simulink model "LinearniUpravljanje"  (R2018a)
settings: Solver=VariableStepAuto  StartTime=0.0  StopTime=15  RelTol=1e-3  EnableMultiTasking=on
values from neighbouring files (symbols this model uses):
  a11 = double(subs(diff(f1,wm),[wm id iq u1 mh],[wmn idn iqn u1n mhn]))    [Linearizacija.m]
  a12 = double(subs(diff(f1,id),[wm id iq u1 mh],[wmn idn iqn u1n mhn]))    [Linearizacija.m]
  a13 = double(subs(diff(f1,iq),[wm id iq u1 mh],[wmn idn iqn u1n mhn]))    [Linearizacija.m]
  a21 = double(subs(diff(f2,wm),[wm id iq u1 mh],[wmn idn iqn u1n mhn]))    [Linearizacija.m]
  a22 = double(subs(diff(f2,id),[wm id iq u1 mh],[wmn idn iqn u1n mhn]))    [Linearizacija.m]
  a23 = double(subs(diff(f2,iq),[wm id iq u1 mh],[wmn idn iqn u1n mhn]))    [Linearizacija.m]
  a31 = double(subs(diff(f3,wm),[wm id iq u1 mh],[wmn idn iqn u1n mhn]))    [Linearizacija.m]
  a32 = double(subs(diff(f3,id),[wm id iq u1 mh],[wmn idn iqn u1n mhn]))    [Linearizacija.m]
  a33 = double(subs(diff(f3,iq),[wm id iq u1 mh],[wmn idn iqn u1n mhn]))    [Linearizacija.m]
  b11 = double(subs(diff(f1,u1),[wm id iq u1 mh],[wmn idn iqn u1n mhn]))    [Linearizacija.m]
  b12 = double(subs(diff(f1,mh),[wm id iq u1 mh],[wmn idn iqn u1n mhn]))    [Linearizacija.m]
  b21 = double(subs(diff(f2,u1),[wm id iq u1 mh],[wmn idn iqn u1n mhn]))    [Linearizacija.m]
  b22 = double(subs(diff(f2,mh),[wm id iq u1 mh],[wmn idn iqn u1n mhn]))    [Linearizacija.m]
  b31 = double(subs(diff(f3,u1),[wm id iq u1 mh],[wmn idn iqn u1n mhn]))    [Linearizacija.m]
  b32 = double(subs(diff(f3,mh),[wm id iq u1 mh],[wmn idn iqn u1n mhn]))    [Linearizacija.m]
  idn = Odgovor(2)    [nominale.m]
  iqn = Odgovor(3)    [nominale.m]
  nn = 3000    [Podaci.m]    (also in Podaci.mat; nominale.m)
  u1n = Odgovor(1)    [nominale.m]
  wmn = nn*pi/30    (= 314.159265359)    [nominale.m]
libraries: simulink x1
settings Model: Creator=Bane  LastModifiedBy=lakim
settings DataIOCC: LimitDataPoints=on
settings OptimizationCC: LifeSpan=inf
settings DebuggingCC: AllowSymbolicDim=off  SFUnexpectedBacktrackingDiag=warning  SFNoUnconditionalDefaultTransitionDiag=warning  SFExecutionAtInitializationDiag=none
settings ModelReferenceCC: PropagateSignalLabelsOutOfModel=off
settings CodeAppCC: StateflowObjectComments=on
settings GRTTargetCC: TargetLangStandard=C89/C90 (ANSI)
settings ConfigComp: CovMetricSettings=dw  CovHtmlReporting=on  CovSaveCumulativeToWorkspaceVar=on  CovSaveSingleToWorkspaceVar=on  CovExternalEMLEnable=off

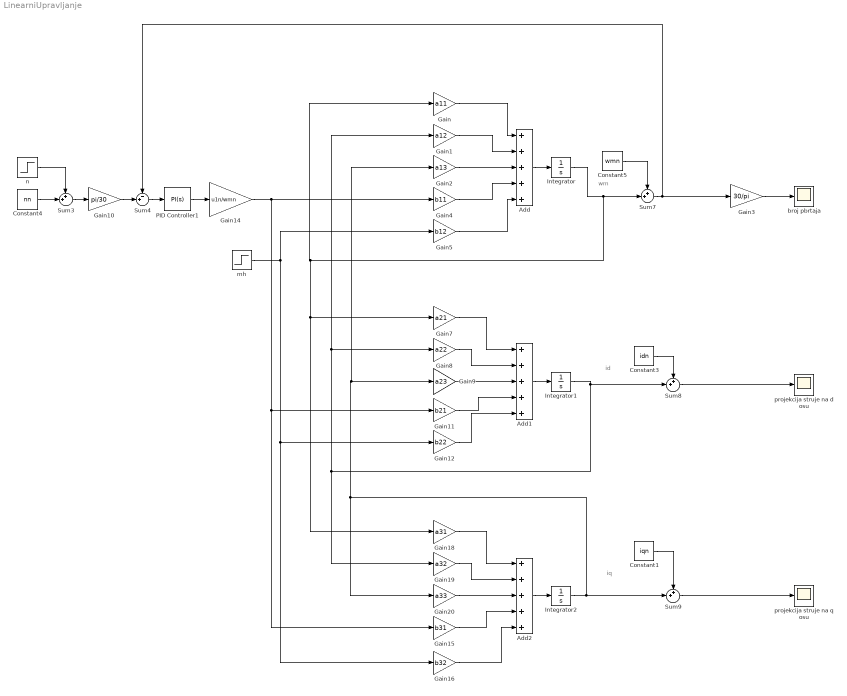
== system LinearniUpravljanje ==
  note: wm
  note: iq
  note: id
  Add : Sum  Inputs=+++++
  Add1 : Sum  Inputs=+++++
  Add2 : Sum  Inputs=+++++
  Constant1 : Constant  Value=iqn
  Constant3 : Constant  Value=idn
  Constant4 : Constant  Value=nn
  Constant5 : Constant  Value=wmn
  Gain : Gain  Gain=a11
  Gain1 : Gain  Gain=a12
  Gain10 : Gain  Gain=pi/30
  Gain11 : Gain  Gain=b21
  Gain12 : Gain  Gain=b22
  Gain14 : Gain  Gain=u1n/wmn
  Gain15 : Gain  Gain=b31
  Gain16 : Gain  Gain=b32
  Gain18 : Gain  Gain=a31
  Gain19 : Gain  Gain=a32
  Gain2 : Gain  Gain=a13
  Gain20 : Gain  Gain=a33
  Gain3 : Gain  Gain=30/pi
  Gain4 : Gain  Gain=b11
  Gain5 : Gain  Gain=b12
  Gain7 : Gain  Gain=a21
  Gain8 : Gain  Gain=a22
  Gain9 : Gain  Gain=a23
  Integrator : Integrator
  Integrator1 : Integrator
  Integrator2 : Integrator
  PID Controller1 : simulink/Continuous/PID Controller  Controller=PI  TimeDomain=Continuous-time  SampleTime=-1  IntegratorMethod=Forward Euler  FilterMethod=Forward Euler  Form=Parallel  UseFilter=on  ControllerParametersSource=internal  P=5  I=65  D=0  N=100  InitialConditionSource=internal  InitialConditionForIntegrator=0  InitialConditionForFilter=0  ExternalReset=none  LimitOutput=off  UpperSaturationLimit=inf  LowerSaturationLimit=-inf  LinearizeAsGain=on  AntiWindupMode=none  Kb=1  TrackingMode=off  Kt=1  PParamMin=[]  PParamMax=[]  IParamMin=[]  IParamMax=[]  DParamMin=[]  DParamMax=[]  NParamMin=[]  NParamMax=[]  KbParamMin=[]  KbParamMax=[]  KtParamMin=[]  KtParamMax=[]  POutMin=[]  POutMax=[]  IOutMin=[]  IOutMax=[]  DOutMin=[]  DOutMax=[]  NOutMin=[]  NOutMax=[]  KbOutMin=[]  KbOutMax=[]  KtOutMin=[]  KtOutMax=[]  IntegratorOutMin=[]  IntegratorOutMax=[]  FilterOutMin=[]  FilterOutMax=[]  SumOutMin=[]  SumOutMax=[]  SumI1OutMin=[]  SumI1OutMax=[]  SumI2OutMin=[]  SumI2OutMax=[]  SumI3OutMin=[]  SumI3OutMax=[]  SumDOutMin=[]  SumDOutMax=[]  SaturationOutMin=[]  SaturationOutMax=[]  IntegratorContinuousStateAttributes=''  IntegratorStateMustResolveToSignalObject=off  IntegratorRTWStateStorageClass=Auto  FilterContinuousStateAttributes=''  FilterStateMustResolveToSignalObject=off  FilterRTWStateStorageClass=Auto  DifferentiatorICPrevScaledInput=0  DifferentiatorOutMin=[]  DifferentiatorOutMax=[]  FilterDiffOutCoefMin=[]  FilterDiffOutCoefMax=[]  SumDenOutMin=[]  SumDenOutMax=[]  SumNumOutMin=[]  SumNumOutMax=[]  ReciprocalOutMin=[]  ReciprocalOutMax=[]  DivideOutMin=[]  DivideOutMax=[]  TunerSelectOption=Transfer Function Based (PID Tuner App)
  Sum{3,7..9} (4 alike) : Sum  Inputs=++|
  Sum4 : Sum  Inputs=-+|
  broj pbrtaja : Scope
  mh : Step  Time=6  After=0.3  SampleTime=0
  n : Step  Time=3  After=100  SampleTime=0
  projekcija struje na d osu : Scope
  projekcija struje na q osu : Scope
  wires:
  Gain4/1 -> Add/4
  Gain5/1 -> Add/5
  Gain18/1 -> Add2/1
  Gain2/1 -> Add/3
  Add2/1 -> Integrator2/1
  Integrator1/1 -> Sum8/2, Gain19/1, Gain8/1, Gain1/1
  Gain7/1 -> Add1/1
  Gain9/1 -> Add1/3
  Gain20/1 -> Add2/3
  Gain19/1 -> Add2/2
  Add/1 -> Integrator/1
  Gain/1 -> Add/1
  Gain8/1 -> Add1/2
  Gain1/1 -> Add/2
  Add1/1 -> Integrator1/1
  Integrator2/1 -> Gain2/1, Gain9/1, Gain20/1, Sum9/2
  Gain15/1 -> Add2/4
  Gain16/1 -> Add2/5
  mh/1 -> Gain5/1, Gain16/1, Gain12/1
  Gain11/1 -> Add1/4
  Gain12/1 -> Add1/5
  Integrator/1 -> Gain18/1, Gain7/1, Gain/1, Sum7/2
  Constant5/1 -> Sum7/1
  Constant3/1 -> Sum8/1
  Constant1/1 -> Sum9/1
  Sum7/1 -> Gain3/1, Sum4/1
  Sum8/1 -> projekcija struje na d osu/1
  Sum9/1 -> projekcija struje na q osu/1
  Gain3/1 -> broj pbrtaja/1
  Gain14/1 -> Gain15/1, Gain11/1, Gain4/1
  Constant4/1 -> Sum3/2
  Sum3/1 -> Gain10/1
  n/1 -> Sum3/1
  Sum4/1 -> PID Controller1/1
  PID Controller1/1 -> Gain14/1
  Gain10/1 -> Sum4/2
